simulink model "constraints_comparison_A_4D_v2"  (R2016a)
settings: Solver=ode4  StartTime=0.0  StopTime=total_time  FixedStep=0.0001  RelTol=1e-3
InitFcn:
  | % clear
  | % clc
undefined symbols (not defined in the file or in its folder): acm_aero_model, acm_T_N, breakpoints1, Cm0, Cmde, Cmq, comp_feedback, constraint_type, dail, de, dele, dele_trim, drud, Fr_mp_1, Fr_mp_2, Fr_rp_1, Fr_rp_2, ini_acm_de_deg, ini_acm_p_deg_per_s, ini_acm_phi_deg, ini_acm_psi_deg, ini_acm_q_deg_per_s, ini_acm_r_deg_per_s, ini_acm_theta_deg, ini_cmp_de_deg, ini_rig_p_deg_per_s, ini_rig_phi_deg, ini_rig_psi_deg, ini_rig_q_deg_per_s, ini_rig_r_deg_per_s, ini_rig_theta_deg, input_type, K1_svo_acm, K1_svo_cmp, K2_svo_acm, K2_svo_cmp, La, Ma, max_defl_sat_acm, max_defl_sat_cmp, max_rate_sat, max_rate_sat_acm, max_rate_sat_cmp, Na, radius, sigbuilder_block, simstop, theta_trim, thrust_trim, windspeed, Xa, Ya, Za
libraries: aerolibconvert2 x119, simulink x42, aerolibtransform2 x19, vrlib x2
(part 4 of 6)

== system constraints_comparison_A_4D_v2/Subsystem14/Compensator servo model4/kinematic ==
  note: If position saturation limit is reached, rate integration is reset
  rate_dot : Inport
  Angle Conversion : aerolibconvert2/Angle Conversion  IU=deg  OU=rad
  Compare To Zero : simulink/Logic and Bit Operations/Compare To Zero  relop=>  OutDataTypeStr=boolean  ZeroCross=off
  Compare To Zero1 : simulink/Logic and Bit Operations/Compare To Zero  relop=<  OutDataTypeStr=boolean  ZeroCross=off
  Compare To Zero2 : simulink/Logic and Bit Operations/Compare To Zero  relop=>  OutDataTypeStr=boolean  ZeroCross=off
  Compare To Zero3 : simulink/Logic and Bit Operations/Compare To Zero  relop=<  OutDataTypeStr=boolean  ZeroCross=off
  Logical Operator : Logic  Operator=OR  AllPortsSameDT=off  OutDataTypeStr=boolean
  Logical Operator1 : Logic  AllPortsSameDT=off  OutDataTypeStr=boolean
  Logical Operator2 : Logic  AllPortsSameDT=off  OutDataTypeStr=boolean
  ini_cmp_de_deg : Constant  Value=ini_cmp_de_deg
  pos : Integrator  InitialConditionSource=external  LimitOutput=on  UpperSaturationLimit=max_defl_sat_cmp  LowerSaturationLimit=-max_defl_sat_cmp  ShowSaturationPort=on  ZeroCross=off
  rate : Integrator  ExternalReset=level hold  UpperSaturationLimit=max_rate_sat  LowerSaturationLimit=-max_rate_sat  ZeroCross=off
  de : Outport
  de_dot : Outport  Port=2
  wires:
  Angle Conversion/1 -> pos/2
  ini_cmp_de_deg/1 -> Angle Conversion/1
  pos/2 -> Compare To Zero2/1, Compare To Zero3/1
  Compare To Zero3/1 -> Logical Operator2/2
  Compare To Zero1/1 -> Logical Operator2/1
  Logical Operator2/1 -> Logical Operator/2
  Compare To Zero2/1 -> Logical Operator1/2
  rate/1 -> pos/1, de_dot/1, Compare To Zero/1, Compare To Zero1/1
  pos/1 -> de/1
  rate_dot/1 -> rate/1
  Logical Operator1/1 -> Logical Operator/1
  Logical Operator/1 -> rate/2
  Compare To Zero/1 -> Logical Operator1/1

== system constraints_comparison_A_4D_v2/Subsystem14/Hawk servo model/kinematic ==
  note: If position saturation limit is reached, rate integration is reset
  rate_dot : Inport
  Angle Conversion : aerolibconvert2/Angle Conversion  IU=deg  OU=rad
  Compare To Zero : simulink/Logic and Bit Operations/Compare To Zero  relop=>  OutDataTypeStr=boolean  ZeroCross=off
  Compare To Zero1 : simulink/Logic and Bit Operations/Compare To Zero  relop=<  OutDataTypeStr=boolean  ZeroCross=off
  Compare To Zero2 : simulink/Logic and Bit Operations/Compare To Zero  relop=>  OutDataTypeStr=boolean  ZeroCross=off
  Compare To Zero3 : simulink/Logic and Bit Operations/Compare To Zero  relop=<  OutDataTypeStr=boolean  ZeroCross=off
  Linear aero model trim (higher accuracy) : Constant  Value=1.1658924813874*pi/180
  Linear aero model trim (higher accuracy)1 : Constant  Value=4.4011
  Logical Operator : Logic  Operator=OR  AllPortsSameDT=off  OutDataTypeStr=boolean
  Logical Operator1 : Logic  AllPortsSameDT=off  OutDataTypeStr=boolean
  Logical Operator2 : Logic  AllPortsSameDT=off  OutDataTypeStr=boolean
  ini_acm_de_deg : Constant  Value=ini_acm_de_deg
  pos : Integrator  InitialConditionSource=external  LimitOutput=on  UpperSaturationLimit=max_defl_sat_acm  LowerSaturationLimit=-max_defl_sat_acm  ShowSaturationPort=on  ZeroCross=off
  rate : Integrator  ExternalReset=level hold  UpperSaturationLimit=max_rate_sat  LowerSaturationLimit=-max_rate_sat  ZeroCross=off
  de : Outport
  de_dot : Outport  Port=2
  wires:
  Compare To Zero/1 -> Logical Operator1/1
  Logical Operator/1 -> rate/2
  Logical Operator1/1 -> Logical Operator/1
  rate_dot/1 -> rate/1
  pos/1 -> de/1
  rate/1 -> Compare To Zero1/1, Compare To Zero/1, de_dot/1, pos/1
  Compare To Zero2/1 -> Logical Operator1/2
  Logical Operator2/1 -> Logical Operator/2
  Compare To Zero1/1 -> Logical Operator2/1
  Compare To Zero3/1 -> Logical Operator2/2
  pos/2 -> Compare To Zero3/1, Compare To Zero2/1
  Linear aero model trim (higher accuracy)/1 -> ?
  ini_acm_de_deg/1 -> Angle Conversion/1
  Angle Conversion/1 -> pos/2

== matlab function constraints_comparison_A_4D_v2/Subsystem14/MATLAB Function1 ==
  data: A2 input; A22 output
function A22 = fcn(A2)

A22 = [ A2(1,1)
        A2(2,1)
        A2(3,1)
        A2(1,2)
        A2(2,2)
        A2(3,2)
        A2(1,3)
        A2(2,3)
        A2(3,3) ];

== matlab function constraints_comparison_A_4D_v2/Subsystem14/Equations of Motion ==
  data: Ac output size=[3,3]; Ar output size=[3,3]; Aa output size=[3,3]; Am output size=[3,3]; Alc output size=[3,3]; Al output size=[3,3]; qc input size=[7,1]; qc_dot_dot output size=[7,1]; qr input size=[7,1]; qa input size=[7,1]; qm input size=[7,1]; qlc input size=[7,1]; ql input size=[7,1]; qc_dot input size=[7,1]; qr_dot input size=[7,1]; qa_dot input size=[7,1]; qm_dot input size=[7,1]; qlc_dot input size=[7,1]; ql_dot input size=[7,1]; F_c input size=[3,1]; M_dash_c input size=[3,1]; qr_dot_dot output size=[7,1]; qa_dot_dot output size=[7,1]; qa_dot_dot2 output size=[3,1]; F_a input size=[3,1]; M_dash_a input size=[3,1]; qm_dot_dot output size=[7,1]; qlc_dot_dot output size=[7,1]; ql_dot_dot output size=[7,1]; RF output; RF_arm output; qa_dot2 output; reaction_forces_lc output; reaction_moments_lc output; reaction_forces_lc_body output; reaction_moments_lc_body output; reaction_forces_a output; reaction_moments_a output; M_dash_l input; Cq_transpose_lc_reaction output
function [Ac,Ar,Aa,Am,Alc,Al,qc_dot_dot,qr_dot_dot,qa_dot_dot,qa_dot_dot2,qm_dot_dot,qlc_dot_dot,ql_dot_dot,RF,RF_arm,qa_dot2,reaction_forces_lc,reaction_moments_lc,reaction_forces_lc_body,reaction_moments_lc_body,reaction_forces_a,reaction_moments_a,Cq_transpose_lc_reaction] = fcn(qc,qr,qa,qm,qlc,ql,qc_dot,qr_dot,qa_dot,qm_dot,qlc_dot,ql_dot,F_c,M_dash_c,F_a,M_dash_a,M_dash_l)

g = 9.81;

%% Compensator properties

m_c = 3.912; % 3.111; % kg
Ixx_c = 0.06524; % kg.m^2
Iyy_c = 0.04421; % kg.m^2
Izz_c = 0.04423; % kg.m^2
Ixy_c = 0; % 9.607E-7; % kg.m^2
Ixz_c = 0; % -1.514E-4; % kg.m^2
Iyz_c = 0; % 1.612E-7; % kg.m^2

% Position of body axes origin (c.g. position) relative to inertial axes origin in body frame of reference
uc0 = [ -0.38-0.3*0
        0.0
        0.0  ];

%% Arm properties

% m_r = 3.6468; % kg
% Ixx_r = 0.09145; % kg.m^2
% Iyy_r = 0.7581*1.04708; % kg.m^2
% Izz_r = 0.6688; % kg.m^2
% Ixy_r = 0; % -6.265E-4; % kg.m^2
% Ixz_r = 0; % 0.1635; % kg.m^2
% Iyz_r = 0; % -2.288E-4; % kg.m^2
% 
% % Position of body axes origin (c.g. position) relative to inertial axes origin in body frame of reference
% ur0 = [ 0.2615
%         0.0
%         0.109  ];

%% New arm modified for load cell (estimated using Autodesk Inventor)

m_r = 2.898; % kg
Ixx_r = 0.113; % kg.m^2
Iyy_r = 0.625; % kg.m^2
Izz_r = 0.513; % kg.m^2
Ixy_r = 0; % -6.265E-4; % kg.m^2
Ixz_r = 0; % 0.1635; % kg.m^2
Iyz_r = 0; % -2.288E-4; % kg.m^2

% Position of body axes origin (c.g. position) relative to inertial axes origin in body frame of reference
ur0 = [ 0.129
        0.0
        0.178  ]; % Remember to change integrator initial conditions
    
%% T-tail arm modified for load cell (estimated using Autodesk Inventor)

% m_r = 3.237; % kg
% Ixx_r = 0.135; % kg.m^2
% Iyy_r = 0.768; % kg.m^2
% Izz_r = 0.634; % kg.m^2
% Ixy_r = 0; % -6.265E-4; % kg.m^2
% Ixz_r = 0; % 0.1635; % kg.m^2
% Iyz_r = 0; % -2.288E-4; % kg.m^2
% 
% % Position of body axes origin (c.g. position) relative to inertial axes origin in body frame of reference
% ur0 = [ 0.169
%         0.0
%         0.219  ]; % Remember to change integrator initial conditions

%% Aircraft properties (Hawk)

m_a = 1.970; % 1.645; % kg
Ixx_a = 0.008083; % 0.00959; % kg.m^2
Iyy_a = 0.038; %0.047642; % 0.044; % kg.m^2
Izz_a = 0.061206; % 0.0507; % kg.m^2
Ixy_a = 0; % kg.m^2
Ixz_a = 0; % kg.m^2
Iyz_a = 0; % kg.m^2

% Position of body axes origin (c.g. position) relative to inertial axes origin in body frame of reference
ua0 = [ 0.8
        0.0
        0.0  ];
% %% Aircraft properties (T-tail)
% 
% m_a = 2.5; % kg (scaled mass = 1.87 kg, increased to 2.5 kg as estimated manufactured mass)
% Ixx_a = 0.0228; % kg.m^2
% Iyy_a = 0.161; % 0.044; % kg.m^2
% Izz_a = 0.181; % 0.0507; % kg.m^2
% Ixy_a = 0; % kg.m^2
% Ixz_a = 0; % kg.m^2
% Iyz_a = 0; % kg.m^2
% 
% % Position of body axes origin (c.g. position) relative to inertial axes origin in body frame of reference
% ua0 = [ 0.95
%         0.0
%         0.0  ];
    
%% Back added mass properties

m_m = 2.0; % kg
Ixx_m = 0.0284; % kg.m^2
Iyy_m = 0.0284; % 0.044; % kg.m^2
Izz_m = 0.0284; % 0.0507; % kg.m^2
Ixy_m = 0; % kg.m^2
Ixz_m = 0; % kg.m^2
Iyz_m = 0; % kg.m^2

% Position of body axes origin (c.g. position) relative to inertial axes origin in body frame of reference
um0 = [ -0.672
        0.0
        0.0  ];
    
%% Load cell properties (estimated using Autodesk Inventor)

m_lc = 0.1; % kg
Ixx_lc = 0.0000426; % kg.m^2
Iyy_lc = 0.0000426; % kg.m^2
Izz_lc = 0.0000179; % kg.m^2
Ixy_lc = 0; % kg.m^2
Ixz_lc = 0; % kg.m^2
Iyz_lc = 0; % kg.m^2

% Position of body axes origin (c.g. position) relative to inertial axes origin in body frame of reference
ulc0 = [ 0.8
        0.0
        0.3183  ]; %0.08825
    
%% Link (load cell to aircraft) properties (estimated using Autodesk Inventor)

m_l = 0.455; % kg
Ixx_l = 0.00320; % kg.m^2
Iyy_l = 0.00320; % kg.m^2
Izz_l = 0.0000895; % kg.m^2
Ixy_l = 0; % kg.m^2
Ixz_l = 0; % kg.m^2
Iyz_l = 0; % kg.m^2

% Position of body axes origin (c.g. position) relative to inertial axes origin in body frame of reference
ul0 = [ 0.8
        0.0
        0.1433  ]; %0.03975

%% Input position and attitude vectors

Rc1 = qc(1);
Rc2 = qc(2);
Rc3 = qc(3);
qc0 = qc(4);
qc1 = qc(5);
qc2 = qc(6);
qc3 = qc(7);

Rr1 = qr(1);
Rr2 = qr(2);
Rr3 = qr(3);
qr0 = qr(4);
qr1 = qr(5);
qr2 = qr(6);
qr3 = qr(7);

Ra1 = qa(1);
Ra2 = qa(2);
Ra3 = qa(3);
qa0 = qa(4);
qa1 = qa(5);
qa2 = qa(6);
qa3 = qa(7);

Rm1 = qm(1);
Rm2 = qm(2);
Rm3 = qm(3);
qm0 = qm(4);
qm1 = qm(5);
qm2 = qm(6);
qm3 = qm(7);

Rlc1 = qlc(1);
Rlc2 = qlc(2);
Rlc3 = qlc(3);
qlc0 = qlc(4);
qlc1 = qlc(5);
qlc2 = qlc(6);
qlc3 = qlc(7);

Rl1 = ql(1);
Rl2 = ql(2);
Rl3 = ql(3);
ql0 = ql(4);
ql1 = ql(5);
ql2 = ql(6);
ql3 = ql(7);

%% Input linear and angular velocity vectors

Rc1_dot = qc_dot(1);
Rc2_dot = qc_dot(2);
Rc3_dot = qc_dot(3);
qc0_dot = qc_dot(4);
qc1_dot = qc_dot(5);
qc2_dot = qc_dot(6);
qc3_dot = qc_dot(7);

Rr1_dot = qr_dot(1);
Rr2_dot = qr_dot(2);
Rr3_dot = qr_dot(3);
qr0_dot = qr_dot(4);
qr1_dot = qr_dot(5);
qr2_dot = qr_dot(6);
qr3_dot = qr_dot(7);

Ra1_dot = qa_dot(1);
Ra2_dot = qa_dot(2);
Ra3_dot = qa_dot(3);
qa0_dot = qa_dot(4);
qa1_dot = qa_dot(5);
qa2_dot = qa_dot(6);
qa3_dot = qa_dot(7);

Rm1_dot = qm_dot(1);
Rm2_dot = qm_dot(2);
Rm3_dot = qm_dot(3);
qm0_dot = qm_dot(4);
qm1_dot = qm_dot(5);
qm2_dot = qm_dot(6);
qm3_dot = qm_dot(7);

Rlc1_dot = qlc_dot(1);
Rlc2_dot = qlc_dot(2);
Rlc3_dot = qlc_dot(3);
qlc0_dot = qlc_dot(4);
qlc1_dot = qlc_dot(5);
qlc2_dot = qlc_dot(6);
qlc3_dot = qlc_dot(7);

Rl1_dot = ql_dot(1);
Rl2_dot = ql_dot(2);
Rl3_dot = ql_dot(3);
ql0_dot = ql_dot(4);
ql1_dot = ql_dot(5);
ql2_dot = ql_dot(6);
ql3_dot = ql_dot(7);

%% Transformation matrices
   
Ec = [  -qc1     qc0      -qc3     qc2
        -qc2     qc3      qc0      -qc1
        -qc3     -qc2     qc1      qc0  ];
    
E_dashc = [     -qc1     qc0      qc3      -qc2
                -qc2     -qc3     qc0      qc1
                -qc3     qc2      -qc1     qc0  ];
        
Er = [  -qr1     qr0      -qr3     qr2
        -qr2     qr3      qr0      -qr1
        -qr3     -qr2     qr1      qr0  ];
        
E_dashr = [     -qr1     qr0      qr3      -qr2
                -qr2     -qr3     qr0      qr1
                -qr3     qr2      -qr1     qr0  ];
            
Ea = [  -qa1     qa0      -qa3     qa2
        -qa2     qa3      qa0      -qa1
        -qa3     -qa2     qa1      qa0  ];
    
E_dasha = [     -qa1     qa0      qa3      -qa2
                -qa2     -qa3     qa0      qa1
                -qa3     qa2      -qa1     qa0  ];
            
Em = [  -qm1     qm0      -qm3     qm2
        -qm2     qm3      qm0      -qm1
        -qm3     -qm2     qm1      qm0  ];
    
E_dashm = [     -qm1     qm0      qm3      -qm2
                -qm2     -qm3     qm0      qm1
                -qm3     qm2      -qm1     qm0  ];
            
Elc = [  -qlc1     qlc0      -qlc3     qlc2
        -qlc2     qlc3      qlc0      -qlc1
        -qlc3     -qlc2     qlc1      qlc0  ];
    
E_dashlc = [     -qlc1     qlc0      qlc3      -qlc2
                -qlc2     -qlc3     qlc0      qlc1
                -qlc3     qlc2      -qlc1     qlc0  ];
            
El = [  -ql1     ql0      -ql3     ql2
        -ql2     ql3      ql0      -ql1
        -ql3     -ql2     ql1      ql0  ];
    
E_dashl = [     -ql1     ql0      ql3      -ql2
                -ql2     -ql3     ql0      ql1
                -ql3     ql2      -ql1     ql0  ];
            
Ac = Ec*transpose(E_dashc);

Ar = Er*transpose(E_dashr);

Aa = Ea*transpose(E_dasha);

Am = Em*transpose(E_dashm);

Alc = Elc*transpose(E_dashlc);

Al = El*transpose(E_dashl);
    
%% Mass and inertial matrix (M) of system

% Mass matrix of compensator
Mc_RR = [   m_c	0   0
            0   m_c	0
            0   0   m_c	];

% Mass matrix of arm
Mr_RR = [   m_r	0   0
            0   m_r	0
            0   0   m_r	];
        
% Mass matrix of aircraft model
Ma_RR = [   m_a	0   0
            0   m_a	0
            0   0   m_a	];
        
% Mass matrix of back added mass
Mm_RR = [   m_m	0   0
            0   m_m	0
            0   0   m_m	];
        
% Mass matrix of load cell
Mlc_RR = [   m_lc	0   0
            0   m_lc	0
            0   0   m_lc	];
        
% Mass matrix of link
Ml_RR = [   m_l	0   0
            0   m_l	0
            0   0   m_l	];
        
% Inertial tensor of compensator in body frame of reference about c.g./body axes
Ic = [   Ixx_c	-Ixy_c	-Ixz_c
        -Ixy_c	 Iyy_c	-Iyz_c
        -Ixz_c	-Iyz_c	 Izz_c	];
    
% Inertial tensor of arm in body frame of reference about c.g./body axes
Ir = [   Ixx_r	-Ixy_r	-Ixz_r
        -Ixy_r	 Iyy_r	-Iyz_r
        -Ixz_r	-Iyz_r	 Izz_r	];
    
% Inertial tensor of aircraft model in body frame of reference about c.g./body axes
Ia = [   Ixx_a	-Ixy_a	-Ixz_a
        -Ixy_a	 Iyy_a	-Iyz_a
        -Ixz_a	-Iyz_a	 Izz_a	];
    
% Inertial tensor of back added mass in body frame of reference about c.g./body axes
Im = [   Ixx_m	-Ixy_m	-Ixz_m
        -Ixy_m	 Iyy_m	-Iyz_m
        -Ixz_m	-Iyz_m	 Izz_m	];
    
% Inertial tensor of load cell in body frame of reference about c.g./body axes
Ilc = [  Ixx_lc	-Ixy_lc	-Ixz_lc
        -Ixy_lc	 Iyy_lc	-Iyz_lc
        -Ixz_lc	-Iyz_lc	 Izz_lc	];
    
% Inertial tensor of link in body frame of reference about c.g./body axes
Il = [   Ixx_l	-Ixy_l	-Ixz_l
        -Ixy_l	 Iyy_l	-Iyz_l
        -Ixz_l	-Iyz_l	 Izz_l	];
    
MMc = [  Mc_RR      zeros(3,4)
        zeros(4,3)	transpose(2*E_dashc)*Ic*2*E_dashc	];
    
MMr = [  Mr_RR    	zeros(3,4)
        zeros(4,3)	transpose(2*E_dashr)*Ir*2*E_dashr	];
    
MMa = [  Ma_RR    	zeros(3,4)
        zeros(4,3)	transpose(2*E_dasha)*Ia*2*E_dasha	];
    
MMm = [  Mm_RR    	zeros(3,4)
        zeros(4,3)	transpose(2*E_dashm)*Im*2*E_dashm	];
    
MMlc = [  Mlc_RR    	zeros(3,4)
        zeros(4,3)	transpose(2*E_dashlc)*Ilc*2*E_dashlc	];
    
MMl = [  Ml_RR    	zeros(3,4)
        zeros(4,3)	transpose(2*E_dashl)*Il*2*E_dashl	];
    
M = [   MMc      	zeros(7)    zeros(7)    zeros(7)    zeros(7)    zeros(7)
        zeros(7)	MMr         zeros(7)    zeros(7)    zeros(7)    zeros(7)
        zeros(7)    zeros(7)    MMa         zeros(7)    zeros(7)    zeros(7)
        zeros(7)    zeros(7)    zeros(7)    MMm         zeros(7)    zeros(7)
        zeros(7)    zeros(7)    zeros(7)    zeros(7)    MMlc        zeros(7)
        zeros(7)    zeros(7)    zeros(7)    zeros(7)    zeros(7)    MMl     ];
    
%% Computing external forces matrix QE

% Angular velocity of compensator in body frame of reference
omega_dashc = 2*E_dashc*[	qc0_dot
                            qc1_dot
                            qc2_dot
                            qc3_dot     ];
                
% Angular velocity of rig in body frame of reference
omega_dashr = 2*E_dashr*[	qr0_dot
                            qr1_dot
                            qr2_dot
                            qr3_dot     ];
                
% Angular velocity of aircraft model in body frame of reference
omega_dasha = 2*E_dasha*[	qa0_dot
                            qa1_dot
                            qa2_dot
                            qa3_dot     ];
                        
% Angular velocity of back added mass in body frame of reference
omega_dashm = 2*E_dashm*[	qm0_dot
                            qm1_dot
                            qm2_dot
                            qm3_dot     ];
                        
% Angular velocity of load cell in body frame of reference
omega_dashlc = 2*E_dashlc*[	qlc0_dot
                            qlc1_dot
                            qlc2_dot
                            qlc3_dot     ];
                        
% Angular velocity of link in body frame of reference
omega_dashl = 2*E_dashl*[	ql0_dot
                            ql1_dot
                            ql2_dot
                            ql3_dot     ];
                
% External translational/linear forces on compensator in inertial frame of reference
% Fc1 = 0;
% Fc2 = 0;
% Fc3 = m_c*9.81;
Fc1 = F_c(1);
Fc2 = F_c(2);
Fc3 = F_c(3)+m_c*g;
Fc = [  Fc1
        Fc2
        Fc3     ];
% External moments on compensator in body frame of reference
% Mc1 = 0;
% Mc2 = 0;
% Mc3 = 0;
Mc1 = M_dash_c(1);
Mc2 = M_dash_c(2);
Mc3 = M_dash_c(3);
Mc = [  Mc1
        Mc2
        Mc3     ];

% External translational/linear forces on arm in inertial frame of reference
Fr1 = 0;
Fr2 = 0;
Fr3 = m_r*g;
Fr = [  Fr1
        Fr2
        Fr3     ];
% External moments on arm in body frame of reference
Mr1 = 0;
Mr2 = 0;
Mr3 = 0;
Mr = [  Mr1
        Mr2
        Mr3     ];
    
% External translational/linear forces on aircraft model in inertial frame of reference
% Fa1 = 0;
% Fa2 = 0;
% Fa3 = m_a*9.81;
Fa1 = F_a(1);
Fa2 = F_a(2);
Fa3 = F_a(3)+m_a*g;
Fa = [  Fa1
        Fa2
        Fa3    ];
% External moments on aircraft model in body frame of reference
% Ma1 = 0;
% Ma2 = 0;
% Ma3 = 0;
Ma1 = M_dash_a(1);
Ma2 = M_dash_a(2);
Ma3 = M_dash_a(3);
Ma = [  Ma1
        Ma2
        Ma3     ];
    
% External translational/linear forces on back added mass in inertial frame of reference
Fm1 = 0;
Fm2 = 0;
Fm3 = m_m*g;
Fm = [  Fm1
        Fm2
        Fm3     ];
% External moments on back added mass in body frame of reference
Mm1 = 0;
Mm2 = 0;
Mm3 = 0;
Mm = [  Mm1
        Mm2
        Mm3     ];
    
% External translational/linear forces on load cell in inertial frame of reference
Flc1 = 0;
Flc2 = 0;
Flc3 = m_lc*g;
Flc = [  Flc1
         Flc2
         Flc3     ];
% External moments on load cell in body frame of reference
Mlc1 = 0;
Mlc2 = 0;
Mlc3 = 0;
Mlc = [  Mlc1
         Mlc2
         Mlc3     ];
    
% External translational/linear forces on link in inertial frame of reference
Fl1 = 0;
Fl2 = 0;
Fl3 = m_l*g;
Fl = [  Fl1
        Fl2
        Fl3     ];
% External moments on link in body frame of reference
Ml1 = M_dash_l(1);
Ml2 = M_dash_l(2);
Ml3 = M_dash_l(3);
Ml = [  Ml1
        Ml2
        Ml3     ];

QE_c = [    Fc
            transpose(2*E_dashc)*(Mc-cross(omega_dashc,Ic*omega_dashc))	];
       
QE_r = [    Fr
            transpose(2*E_dashr)*(Mr-cross(omega_dashr,Ir*omega_dashr))	];
        
QE_a = [    Fa
            transpose(2*E_dasha)*(Ma-cross(omega_dasha,Ia*omega_dasha))	];
        
QE_m = [    Fm
            transpose(2*E_dashm)*(Mm-cross(omega_dashm,Im*omega_dashm))	];
        
QE_lc = [    Flc
            transpose(2*E_dashlc)*(Mlc-cross(omega_dashlc,Ilc*omega_dashlc))	];
        
QE_l = [    Fl
            transpose(2*E_dashl)*(Ml-cross(omega_dashl,Il*omega_dashl))	];
        
QE = [  QE_c
        QE_r
        QE_a    
        QE_m
        QE_lc
        QE_l    ];

    
%% Spherical joint constraint for compensator

% Skew symmetric (antisymmetric) matrix
ssc0 = Ac*uc0;
ssc = [	0           -ssc0(3)	ssc0(2)
       	ssc0(3)     0           -ssc0(1)
      	-ssc0(2)	ssc0(1)   	0       ];

Cq_1 = [    eye(3)      ssc*2*Ec     zeros(3,21)    ];

%% Spherical joint constraint for arm

% Skew symmetric (antisymmetric) matrix
ssr0 = Ar*ur0;
ssr = [	0           -ssr0(3)	ssr0(2)
      	ssr0(3)     0           -ssr0(1)
    	-ssr0(2)	ssr0(1)     0       ];

Cq_2 = [    zeros(3,7)  eye(3)  ssr*2*Er    zeros(3,14)  zeros(3,14) ];

%% Attitude constraint between compensator and arm

Cq_3 = [	zeros(4,3)	eye(4)	zeros(4,3)	-eye(4)	zeros(4,14)];

%% Aircraft model position vector constraint to arm/compensator

% Skew symmetric (antisymmetric) matrix
ssa0 = Ac*ua0;
ssa = [	0           -ssa0(3)	ssa0(2)
       	ssa0(3)     0           -ssa0(1)
      	-ssa0(2)	ssa0(1)   	0       ];

Cq_4 = [    zeros(3)  ssa*2*Ec	zeros(3)	zeros(3,4)	eye(3)     zeros(3,4)   zeros(3,7)	];

%% Quaternion unit norm constraint for compensator (constraint for arm and back added mass not required due to constraint Cq_3)

Cq_5 = [    zeros(1,3)  2*qc0   2*qc1   2*qc2   2*qc3   zeros(1,21)     ];

%% Quaternion unit norm constraint for aircraft model

Cq_6 = [    zeros(1,7)  zeros(1,7)  zeros(1,3)  2*qa0   2*qa1   2*qa2   2*qa3   zeros(1,7)  zeros(1,14) ];

%% Spherical joint constraint for back added mass

% Skew symmetric (antisymmetric) matrix
ssm0 = Am*um0;
ssm = [	0           -ssm0(3)	ssm0(2)
       	ssm0(3)     0           -ssm0(1)
      	-ssm0(2)	ssm0(1)   	0       ];
        
Cq_7 = [	zeros(3,21)     eye(3)      ssm*2*Em     ];

%% Attitude constraint between compensator and back added mass

Cq_8 = [	zeros(4,3)      eye(4)      zeros(4,14)     zeros(4,3)      -eye(4)     ];

%% Quaternion constraint for back added mass (not needed if Cq_7 and Cq_8 are in effect)

Cq_9 = [	zeros(1,21)     zeros(1,3)  2*qm0   2*qm1   2*qm2   2*qm3     zeros(1,14) ];

%% Quaternion constraint for arm

Cq_10 = [	zeros(1,7)	zeros(1,3)	2*qr0   2*qr1   2*qr2   2*qr3   zeros(1,14)  zeros(1,14) ];

%% Arm to compensator fixed constraint

% Cq_4 = [    zeros(3)  ssa*2*Ec	zeros(3)	zeros(3,4)	eye(3)     zeros(3,4)   zeros(3,7)	];

% Cq_11 = [	eye(3)  zeros(3,4) -eye(3) zeros(3,4) zeros(3,14) 
%             zeros(4,3)  eye(4)  zeros(4,3)  -eye(4) zeros(4,14)  ];

% Skew symmetric (antisymmetric) matrix
ssc0 = Ar*uc0;
ssc = [	0           -ssc0(3)	ssc0(2)
       	ssc0(3)     0           -ssc0(1)
      	-ssc0(2)	ssc0(1)   	0       ];
    
Cq_11 = [	eye(3)  zeros(3,4) zeros(3) ssc*2*Er zeros(3,14)  zeros(3,14) 
            zeros(4,3)  eye(4)  zeros(4,3)  -eye(4) zeros(4,14)  zeros(4,14) ];
        
%% Quaternion constraint for load cell

Cq_12 = [	zeros(1,7)  zeros(1,7)  zeros(1,14)  zeros(1,3)	2*qlc0   2*qlc1   2*qlc2   2*qlc3  zeros(1,7) ];

%% Quaternion constraint for link

Cq_13 = [	zeros(1,14)   zeros(1,14)  zeros(1,7)  zeros(1,3)	2*ql0   2*ql1   2*ql2   2*ql3  ];

%% Arm to load cell fixed constraint

% Skew symmetric (antisymmetric) matrix
sslc0 = Ar*ulc0;
sslc = [	0           -sslc0(3)	sslc0(2)
       	sslc0(3)     0           -sslc0(1)
      	-sslc0(2)	sslc0(1)   	0       ];

Cq_14 = [	zeros(3)  zeros(3,4) zeros(3) sslc*2*Er zeros(3,14)  eye(3) zeros(3,4) zeros(3,7) 
            zeros(4,7) zeros(4,3)  eye(4) zeros(4,14) zeros(4,3)  -eye(4) zeros(4,7) ];

% Skew symmetric (antisymmetric) matrix
sslc0 = Alc*(ulc0-ur0);
sslc = [	0           -sslc0(3)	sslc0(2)
       	sslc0(3)     0           -sslc0(1)
      	-sslc0(2)	sslc0(1)   	0       ];

Cq_14_2 = [	zeros(3)  zeros(3,4) -eye(3) sslc*2*Elc zeros(3,14)  eye(3) zeros(3,4) zeros(3,7) 
            zeros(4,7) zeros(4,3)  eye(4) zeros(4,14) zeros(4,3)  -eye(4) zeros(4,7) ];
        
%% Link to load cell fixed constraint

% Skew symmetric (antisymmetric) matrix
ssl0 = Alc*ul0;
ssl = [	0           -ssl0(3)	ssl0(2)
       	ssl0(3)     0           -ssl0(1)
      	-ssl0(2)	ssl0(1)   	0       ];

Cq_15 = [	zeros(3)  zeros(3,4) zeros(3,14)  zeros(3,7)  zeros(3) ssl*2*Elc  eye(3) zeros(3,4) 
            zeros(4,7)  zeros(4,21) zeros(4,3)  eye(4) zeros(4,3)  -eye(4) ];
        
%% Load cell to link fixed constraint (DOES NOT WORK)

% Skew symmetric (antisymmetric) matrix
ssl0 = Al*ulc0;
ssl = [	0           -ssl0(3)	ssl0(2)
       	ssl0(3)     0           -ssl0(1)
      	-ssl0(2)	ssl0(1)   	0       ];

Cq_15_2 = [	zeros(3)  zeros(3,4) zeros(3,14)  zeros(3,7)  eye(3) zeros(3,4)  zeros(3) ssl*2*El   
            zeros(4,7)  zeros(4,21) zeros(4,3)  -eye(4) zeros(4,3)  eye(4) ];
        
%% Link to load cell fixed constraint

% Skew symmetric (antisymmetric) matrix
ssl0 = Alc*(ul0-ulc0);
ssl = [	0           -ssl0(3)	ssl0(2)
       	ssl0(3)     0           -ssl0(1)
      	-ssl0(2)	ssl0(1)   	0       ];

Cq_15_3 = [	zeros(3)  zeros(3,4) zeros(3,14)  zeros(3,7)  -eye(3) ssl*2*Elc  eye(3) zeros(3,4) 
            zeros(4,7)  zeros(4,21) zeros(4,3)  eye(4) zeros(4,3)  -eye(4) ];
        
%% Link to aircraft model position fixed constraint

% Skew symmetric (antisymmetric) matrix
ssa0 = Al*ua0;
ssa = [	0           -ssa0(3)	ssa0(2)
       	ssa0(3)     0           -ssa0(1)
      	-ssa0(2)	ssa0(1)   	0       ];

Cq_16 = [    zeros(3,7) zeros(3,7)  eye(3) zeros(3,4)  zeros(3,7) zeros(3,7)  zeros(3) ssa*2*El	];

% Skew symmetric (antisymmetric) matrix
ssa0 = Al*(ua0-ul0);
ssa = [	0           -ssa0(3)	ssa0(2)
       	ssa0(3)     0           -ssa0(1)
      	-ssa0(2)	ssa0(1)   	0       ];

Cq_16_2 = [    zeros(3,7) zeros(3,7)  eye(3) zeros(3,4)  zeros(3,7) zeros(3,7)  -eye(3) ssa*2*El	];

%% Arm pitch and yaw fixed (Remember to disable quaternion contraint for arm (Cq_10))

% Cq_17 = [ zeros(3,7) eye(3) zeros(3,4) zeros(3,28) ]; % Does not completely fix arm, try attitude fix
% Cq_17 = [ zeros(3,7) eye(3)      zeros(3,4) zeros(3,28) 
%           zeros(4,7) zeros(4,3)  eye(4)     zeros(4,28) ];
Cq_17 = [ zeros(4,7) zeros(4,3)  eye(4)     zeros(4,28) ];

%% Rig yaw only constraint (fixing arm c.g. to move in only x and y directions, i.e. no acceleration in z direction)

Cq_18 = [   zeros(1,7) [ 0 0 1 0 0 0 0] zeros(1,7*4) ];
      
%% Rig roll only constraint (fully fix compensator inertial axes position, i.e. zero acceleration in all directions)

Cq_19 = [   0 1 0 zeros(1,4)  zeros(1,7*5)
            0 0 1 zeros(1,4)  zeros(1,7*5)  ];
        
%% Link to aircraft attitude fixed constraint  (Remember to disable quaternion contraint for acm (Cq_6))

Cq_20= [	zeros(4,7)  zeros(4,7) zeros(4,3)  -eye(4) zeros(4,7) zeros(4,7) zeros(4,3)  eye(4) ];
        
%% Computing matrix Cq from constraint equations

% Cq = [  Cq_1 	
%         Cq_2    
%         Cq_3    
%         Cq_4    
%         Cq_5
%         Cq_6
%         Cq_9    ];
    
% With back added mass: include Cq_7 and Cq_8, remove Cq_9
% Without back added mass: include Cq_9, remove Cq_7 and Cq_8

Cq = [  Cq_2
        Cq_6
        Cq_9
        Cq_10
        Cq_11
        Cq_14_2
        Cq_15_3
        Cq_16_2
        %Cq_17
        %Cq_18
        %Cq_19
        %Cq_20
        ];
    
%% Computing matrix QC

% Angular velocity of compensator in inertial frame of reference
omegac = 2*Ec*[     qc0_dot
                    qc1_dot
                    qc2_dot
                    qc3_dot     ];
                
% Angular velocity of arm in inertial frame of reference
omegar = 2*Er*[     qr0_dot
                    qr1_dot
                    qr2_dot
                    qr3_dot     ];
                
% Angular velocity of back added mass in inertial frame of reference
omegam = 2*Em*[     qm0_dot
                    qm1_dot
                    qm2_dot
                    qm3_dot     ];
                
% Angular velocity of load cell in inertial frame of reference
omegalc = 2*Elc*[   qlc0_dot
                    qlc1_dot
                    qlc2_dot
                    qlc3_dot     ];
                
% Angular velocity of link in inertial frame of reference
omegal = 2*El*[     ql0_dot
                    ql1_dot
                    ql2_dot
                    ql3_dot     ];
                
QC_1 = cross(omegac,cross(omegac,Ac*uc0));

QC_2 = cross(omegar,cross(omegar,Ar*ur0));

QC_3 = zeros(4,1);

QC_4 = cross(omegac,cross(omegac,Ac*ua0));

QC_5 = -(2*(qc0_dot)^2+2*(qc1_dot)^2+2*(qc2_dot)^2+2*(qc3_dot)^2);

QC_6 = -(2*(qa0_dot)^2+2*(qa1_dot)^2+2*(qa2_dot)^2+2*(qa3_dot)^2);

QC_7 = cross(omegam,cross(omegam,Am*um0));

QC_8 = zeros(4,1);

QC_9 = -(2*(qm0_dot)^2+2*(qm1_dot)^2+2*(qm2_dot)^2+2*(qm3_dot)^2);

QC_10 = -(2*(qr0_dot)^2+2*(qr1_dot)^2+2*(qr2_dot)^2+2*(qr3_dot)^2);

QC_11 = [   cross(omegar,cross(omegar,Ar*uc0))
            zeros(4,1)  ];
        
QC_12 = -(2*(qlc0_dot)^2+2*(qlc1_dot)^2+2*(qlc2_dot)^2+2*(qlc3_dot)^2);

QC_13 = -(2*(ql0_dot)^2+2*(ql1_dot)^2+2*(ql2_dot)^2+2*(ql3_dot)^2);

QC_14 = [   cross(omegar,cross(omegar,Ar*ulc0))
            zeros(4,1)  ];

QC_14_2 = [   cross(omegalc,cross(omegalc,Alc*(ulc0-ur0)))
            zeros(4,1)  ];
        
QC_15 = [   cross(omegalc,cross(omegalc,Alc*ul0))
            zeros(4,1)  ];
        
QC_15_2 = [ cross(omegal,cross(omegal,Al*ulc0))
            zeros(4,1)  ];  % (DOES NOT WORK)
        
QC_15_3 = [ cross(omegalc,cross(omegalc,Alc*(ul0-ulc0)))
            zeros(4,1)  ];
        
QC_16 = [   cross(omegal,cross(omegal,Al*ua0))  ];

QC_16_2 = [   cross(omegal,cross(omegal,Al*(ua0-ul0)))  ];

% QC_17 = [ zeros(3,1) ];
% QC_17 = [   0
%             0
%             0
%             1
%             0
%             0
%             0   ];
QC_17 = [   0
            0
            0
            0   ];
        
QC_18 = [   0   ];
        
QC_19 = [   zeros(2,1)  ];

QC_20 = [   0
            0
            0
            0   ];

% QC = [  QC_1
%         QC_2
%         QC_3    
%         QC_4    
%         QC_5
%         QC_6
%         QC_9    ];
    
% With back added mass: include QC_7 and QC_8, remove QC_9
% Without back added mass: include QC_9, remove QC_7 and QC_8

QC = [  QC_2
        QC_6
        QC_9
        QC_10
        QC_11
        QC_14_2
        QC_15_3
        QC_16_2
        %QC_17
        %QC_18
        %QC_19
        %QC_20
        ];
    
%% Solving equations of motion

% Use MM below when including back added mass
% MM = [  M   transpose(Cq)
%         Cq  zeros(22)        ];

% Use MM below when not including back added mass
% MM = [  M   transpose(Cq)
%         Cq  zeros(16)        ];

% New MM matrix for load cell update
MM = [  M   transpose(Cq)
        Cq  zeros(size(QC,1))        ]; % zeros(7+3+4-1+2+(-1+7)+(-1+7)+(3)+(4)-1)

QQ = [  QE
        QC  ];
    
qq = MM\QQ;

%% Output acceleration vectors

qc_dot_dot = qq(1:7);
qr_dot_dot = qq(8:14);
qa_dot_dot = qq(15:21);
qm_dot_dot = qq(22:28);
qlc_dot_dot = qq(29:35);
ql_dot_dot = qq(36:42);

% qc_dot_dot = zeros(7,1); % Setting compensator accelerations to always be zero
% qr_dot_dot = zeros(7,1);
% qa_dot_dot(1:3,1) = zeros(3,1);
% qm_dot_dot = zeros(7,1);

% qa_dot_dot2 = [ qa_dot_dot(1:3,1)
%                 2*E_dasha*qa_dot_dot(4:7,1)     ];

qa_dot_dot2 = [ qa_dot_dot(1:3,1)   ];

qa_dot2 = [ qa_dot(1:3,1)
           2*E_dasha*qa_dot(4:7,1)     ];
            
%% Reaction forces and moments

% Use RF below when including back added mass
% RF = transpose(Cq)*qq(29:50);

% Use RF below when not including back added mass
% RF = transpose(Cq)*qq(29:44);
RF = zeros(40,1);

% RF_arm = transpose(Ac)*RF(15:17,1);
RF_arm = 0;

% CqTT = transpose(Cq);
% CqT = CqTT(15:21,11:15);
% lagrange = qq(29:44);

% CqT_lagrange_quart = CqTT(:,14:16)*qq(42:44);
CqT_lagrange_quart = 0;

%% Reaction forces and moments investigation

% R1 = -CqTT(1:7,1:3)*lagrange(1:3,1); % Reaction forces and moments from spherical constraint on compensator
R1 = 0;

%% Load cell reaction forces
Cq_transpose = transpose(Cq);
Cq_transpose_lc = Cq_transpose(29:35,:);
% Cq_transpose_lc_reaction = Cq_transpose_lc(:,21:27); % With Cq_6
Cq_transpose_lc_reaction = Cq_transpose_lc(:,20:26); % Without Cq_6
lagrange_multipliers = qq(43:end); % (7 states)*(6 bodies) = 42 vector size
% lagrange_lc = lagrange_multipliers(21:27); % With Cq_6
lagrange_lc = lagrange_multipliers(20:26); % Without Cq_6

% Cq_transpose_lc = Cq_transpose(29:35,:);
% Cq_transpose_r_reaction = Cq_transpose_lc(:,14:20);
% % lagrange_multipliers = qq(43:end);
% lagrange_r = lagrange_multipliers(14:20);

reaction_loads_lc = -Cq_transpose_lc_reaction*lagrange_lc;
reaction_forces_lc = reaction_loads_lc(1:3); % CORRECT
reaction_moments_lc = 0.5*E_dashlc*reaction_loads_lc(4:7) + cross(omega_dashlc,Ilc*omega_dashlc); % CORRECT
reaction_forces_lc_body = transpose(Alc)*reaction_forces_lc;
reaction_moments_lc_body = reaction_moments_lc;

% reaction_loads_r = -Cq_transpose_r_reaction*lagrange_r;
% reaction_forces_r = reaction_loads_r(1:3); % CORRECT
% reaction_moment_r = 0.5*E_dashr*reaction_loads_r(4:7); % 0.5*E_dashlc*reaction_loads_lc(4:7) + cross(omega_dashlc,Ilc*omega_dashlc); % CORRECT


% moment_r = transpose(2*E_dashr)*(Mr);
% reaction_moment_r = 0.5*E_dashr*moment_r;

constraint_loads = -Cq_transpose_lc*lagrange_multipliers;
constraint_forces = constraint_loads(1:3);

% % % Cq_transpose_l = Cq_transpose(36:42,:);
% % % Cq_transpose_l_reaction = Cq_transpose_l(:,end-2:end);
% % % lagrange_l = lagrange_multipliers(28:30);
% % % reaction_loads_l = -Cq_transpose_l_reaction*lagrange_l;
% % % reaction_forces_l = reaction_loads_l(1:3);

% reaction_forces = reaction_forces_lc;
% reaction_moments = reaction_moments_lc;

%% Aircraft reaction forces

CqT_lagrange = Cq_transpose*lagrange_multipliers;
reaction_loads_a = --CqT_lagrange(15:21);
reaction_forces_a = reaction_loads_a(1:3);
reaction_moments_a = 0.5*E_dasha*reaction_loads_a(4:7) + cross(omega_dasha,Ia*omega_dasha);

== matlab function constraints_comparison_A_4D_v2/Subsystem14/MATLAB Function2 ==
  data: A1 input; A11 output
function A11 = fcn(A1)

A11 = [ A1(1,1)
        A1(2,1)
        A1(3,1)
        A1(1,2)
        A1(2,2)
        A1(3,2)
        A1(1,3)
        A1(2,3)
        A1(3,3) ];

== matlab function constraints_comparison_A_4D_v2/Subsystem14/MATLAB Function3 ==
  data: V0 output size=[1]; qa input size=[7,1]; alpha output size=[1]; beta output; qa_dot input size=[7,1]; w_dot output size=[1]; q output size=[1]; qa_dot_dot input; Vt input; Va output; qa_wind output
function [V0,alpha,beta,w_dot,q,Va,qa_wind] = fcn(qa,qa_dot,qa_dot_dot,Vt)
  
Ra1 = qa(1);
Ra2 = qa(2);
Ra3 = qa(3);
qa0 = qa(4);
qa1 = qa(5);
qa2 = qa(6);
qa3 = qa(7);

Ra1_dot = qa_dot(1);
Ra2_dot = qa_dot(2);
Ra3_dot = qa_dot(3);
qa0_dot = qa_dot(4);
qa1_dot = qa_dot(5);
qa2_dot = qa_dot(6);
qa3_dot = qa_dot(7);

Ra1_dot_dot = qa_dot_dot(1);
Ra2_dot_dot = qa_dot_dot(2);
Ra3_dot_dot = qa_dot_dot(3);
qa0_dot_dot = qa_dot_dot(4);
qa1_dot_dot = qa_dot_dot(5);
qa2_dot_dot = qa_dot_dot(6);
qa3_dot_dot = qa_dot_dot(7);

% Transformation matrices
Ea = [  -qa1     qa0      -qa3     qa2
        -qa2     qa3      qa0      -qa1
        -qa3     -qa2     qa1      qa0  ];
    
E_dasha = [     -qa1     qa0      qa3      -qa2
                -qa2     -qa3     qa0      qa1
                -qa3     qa2      -qa1     qa0  ];

Aa = Ea*transpose(E_dasha);

% Wind tunnel velocity vector
Vtt = [  Vt
         0   
         0   ];

% Velocity vector of aircraft model in inertial frame of reference
Va = [  Ra1_dot
        Ra2_dot
        Ra3_dot	];

% Total velocity vector of aircraft model in body frame of reference
Va_dash = transpose(Aa)*(Va + Vtt);

% Magnitude of total local velocity vector
V0 = sqrt((Va_dash(1))^2+(Va_dash(2))^2+(Va_dash(3))^2);

% Angle of attack
alpha = atan2(Va_dash(3),Va_dash(1));

% Acceleration in body frame
a_dash = transpose(Aa)*[    Ra1_dot_dot
                            Ra2_dot_dot
                            Ra3_dot_dot     ];

% Acceleration in z-direction body frame
w_dot = a_dash(3);

% Sideslip angle [CHECK SIGN]
beta = asin(Va_dash(2)/V0);

% Local angular velocities (body axes)
omega_dasha = 2*E_dasha*[	qa0_dot
                            qa1_dot
                            qa2_dot
                            qa3_dot     ];
                        
% Pitch rate (body axes)
q = omega_dasha(2);

%% Calculating angular rates in wind axes

phi = 0;
theta = alpha;
psi = -beta;

theta1 = psi;
theta2 = theta;
theta3 = phi;

q0 = +sin(theta1/2)*sin(theta2/2)*sin(theta3/2)+cos(theta1/2)*cos(theta2/2)*cos(theta3/2);
q1 = -sin(theta1/2)*sin(theta2/2)*cos(theta3/2)+sin(theta3/2)*cos(theta1/2)*cos(theta2/2);
q2 = +sin(theta1/2)*sin(theta3/2)*cos(theta2/2)+sin(theta2/2)*cos(theta1/2)*cos(theta3/2);
q3 = +sin(theta1/2)*cos(theta2/2)*cos(theta3/2)-sin(theta2/2)*sin(theta3/2)*cos(theta1/2);

% E = [  -q1     q0      -q3     q2
%         -q2     q3      q0      -q1
%         -q3     -q2     q1      q0  ];
%     
% E_dash = [     -q1     q0      q3      -q2
%                 -q2     -q3     q0      q1
%                 -q3     q2      -q1     q0  ];
%             
%  A_b2w = E*transpose(E_dash); % body axes to inertial/wind axes transformation

qa_wind = [ q0
            q1
            q2
            q3	];

== matlab function constraints_comparison_A_4D_v2/Subsystem14/Extracting position vector 4/MATLAB Function ==
  data: u input; y output
function y = fcn(u)
%#codegen

y = [   u(1)
        u(2)
        u(3)    ];

== matlab function constraints_comparison_A_4D_v2/Subsystem14/Subsystem11/MATLAB Function ==
  data: q input; x_ini output; y_ini output; z_ini output
function [x_ini,y_ini,z_ini]= fcn(q)

% Initial position

x = 0.8;
z = 0.3183;%0.08825;

p = [   x
        0
        z   ];

q0 = q(1);
q1 = q(2);
q2 = q(3);
q3 = q(4);

E = [  -q1     q0      -q3     q2
       -q2     q3      q0      -q1
       -q3     -q2     q1      q0  ];
    
E_dash = [     -q1     q0      q3      -q2
               -q2     -q3     q0      q1
               -q3     q2      -q1     q0  ];
           
A = E*transpose(E_dash);

p_in = A*p;

x_ini = p_in(1);
y_ini = p_in(2);
z_ini = p_in(3);

== matlab function constraints_comparison_A_4D_v2/Subsystem14/MATLAB Function6 ==
  data: A3 input; A33 output
function A33 = fcn(A3)

A33 = [ A3(1,1)
        A3(2,1)
        A3(3,1)
        A3(1,2)
        A3(2,2)
        A3(3,2)
        A3(1,3)
        A3(2,3)
        A3(3,3) ];

== matlab function constraints_comparison_A_4D_v2/Subsystem14/Extracting position vector 1/MATLAB Function ==
  data: u input; y output
function y = fcn(u)
%#codegen

y = [   u(1)
        u(2)
        u(3)    ];

== matlab function constraints_comparison_A_4D_v2/Subsystem14/Extracting position vector 2 /MATLAB Function ==
  data: u input; y output
function y = fcn(u)
%#codegen

y = [   u(1)
        u(2)
        u(3)    ];

== matlab function constraints_comparison_A_4D_v2/Subsystem14/Extracting position vector 3/MATLAB Function ==
  data: u input; y output
function y = fcn(u)
%#codegen

y = [   u(1)
        u(2)
        u(3)    ];

== matlab function constraints_comparison_A_4D_v2/Subsystem14/MATLAB Function4 ==
  data: q2 output size=[4,1]; q1 input size=[7,1]
function q2  = fcn(q1)

q2 = q1(4:7,1);
